simulink model "Servo_model_validate"  (R2020a)
settings: Solver=ode5  StartTime=0.0  StopTime=20  FixedStep=0.002  RelTol=1e-3  AbsTol=1e-6
PreLoadFcn:
  | load servo_chstat
values from neighbouring files (symbols this model uses):
  input_change = 0.07    [lab5.m]
  pwm = [-1 -0.961416361416 -0.923076923077 -0.884493284493 -0.846153846154 -0.80757020757 -0.768986568987 -0.730647130647 -0.692307692308 -0.653724053724 -0.615384615385 -0.576800976801 ... (53 elements, 1x53)]    [servo_chstat.mat]
  vpwm = [-172.202819824 -162.381335449 -154.255700684 -146.997290039 -139.415771484 -132.329187012 -124.019897461 -116.524291992 -108.629003906 -99.2582519531 -92.2202270508 -84.5235351562 ... (53 elements, 1x53)]    [servo_chstat.mat]
libraries: simulink x1
settings Model: ExtModeTrigDuration=12000  ExtModeTrigLevel=0.400000  Creator=jims  LastModifiedBy=ariana
settings SolverCC: AutoScaleAbsTol=off
settings DataIOCC: ExternalInput=[]  InitialState=[]  MaxDataPoints=5000  SaveFormat=Array  SignalLoggingSaveFormat=ModelDataLogs  SaveOutput=off  SaveTime=off  ReturnWorkspaceOutputs=off  SignalLoggingName=sigsOut
settings OptimizationCC: BooleanDataType=off  ExpressionDepthLimit=2147483647  InitFltsAndDblsToZero=on  LifeSpan=inf
settings DebuggingCC: SaveWithParameterizedLinksMsg=none  UnderspecifiedInitializationDetection=Classic  MergeDetectMultiDrivingBlocksExec=none  SignalResolutionControl=TryResolveAllWithWarning  MultiTaskDSMMsg=warning  MultiTaskCondExecSysMsg=none  IntegerOverflowMsg=none  FcnCallInpInsideContextMsg=warning  StateNameClashWarn=warning  SFUnexpectedBacktrackingDiag=warning  SFNoUnconditionalDefaultTransitionDiag=warning  SFExecutionAtInitializationDiag=none  IntegerSaturationMsg=none  ArithmeticOperatorsInVariantConditions=warning
settings HardwareCC: ProdBitPerPointer=32  ProdBitPerSizeT=32  ProdBitPerPtrDiffT=32  ProdLargestAtomicFloat=None  ProdIntDivRoundTo=Undefined  ProdEndianess=Unspecified  ProdWordSize=32  ProdHWDeviceType=32-bit Generic  TargetUnknown=on
settings ModelReferenceCC: PropagateSignalLabelsOutOfModel=off
settings SFSimCC: SimUseLocalCustomCode=off  CustomCodeUndefinedFunction=UseInterfaceOnly
settings RTWCC: SystemTargetFile=rtwin.tlc  TemplateMakefile=rtwintmf  RTWUseLocalCustomCode=off
settings CodeAppCC: StateflowObjectComments=on
settings TargetCC: TargetFcnLib=ansi_tfl_tmw.mat  ModelReferenceCompliant=off  CompOptLevelCompliant=off
settings ConfigComp: CovMetricSettings=dw  CovHtmlReporting=on  CovSaveCumulativeToWorkspaceVar=on  CovSaveSingleToWorkspaceVar=on  CovExternalEMLEnable=off

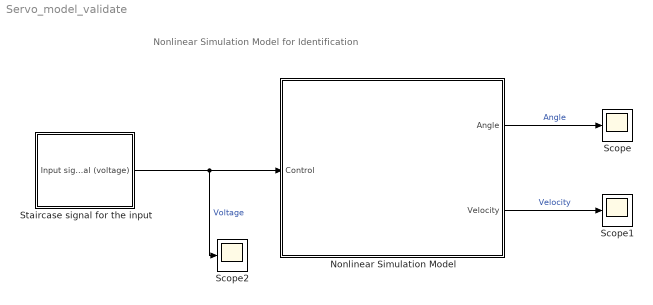
== system Servo_model_validate ==
  note: Nonlinear Simulation Model for Identification
  Nonlinear Simulation Model : Subsystem
  Scope : Scope
  Scope1 : Scope
  Scope2 : Scope
  Staircase signal for the input : Subsystem
  wires:
  Nonlinear Simulation Model/1(Angle) -> Scope/1  "Angle"
  Nonlinear Simulation Model/2(Velocity) -> Scope1/1  "Velocity"
  Staircase signal for the input/1(Input signal (voltage)) -> Scope2/1, Nonlinear Simulation Model/1(Control)  "Voltage"

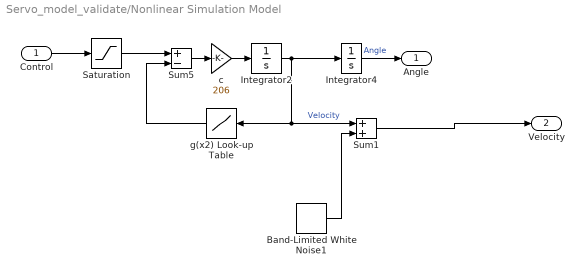
== system Servo_model_validate/Nonlinear Simulation Model ==
  Control : Inport
  Band-Limited White Noise1 : simulink/Sources/Band-Limited White Noise  Cov=[0.001]  Ts=0.02  seed=[23341]
  Integrator2 : Integrator
  Integrator4 : Integrator
  Saturation : Saturate  UpperLimit=1  LowerLimit=-1
  Sum1 : Sum  InputSameDT=on  SaturateOnIntegerOverflow=on  OutDataTypeStr=Inherit: Same as first input
  Sum5 : Sum  Inputs=+-  InputSameDT=on  SaturateOnIntegerOverflow=on  OutDataTypeStr=Inherit: Same as first input
  c : Gain  Gain=206  SaturateOnIntegerOverflow=on  OutDataTypeStr=Inherit: Same as input  ParamDataTypeStr=Inherit: Same as input
  g(x2) Look-up Table : Lookup  InputValues=vpwm  Table=pwm  SaturateOnIntegerOverflow=on
  Angle : Outport  InitialOutput=0  VectorParamsAs1DForOutWhenUnconnected=off
  Velocity : Outport  Port=2  InitialOutput=0  VectorParamsAs1DForOutWhenUnconnected=off
  wires:
  Sum5/1 -> c/1
  g(x2) Look-up Table/1 -> Sum5/2
  Integrator2/1 -> Integrator4/1, g(x2) Look-up Table/1, Sum1/1  "Velocity"
  Integrator4/1 -> Angle/1  "Angle"
  c/1 -> Integrator2/1
  Control/1 -> Saturation/1
  Saturation/1 -> Sum5/1
  Sum1/1 -> Velocity/1
  Band-Limited White Noise1/1 -> Sum1/2

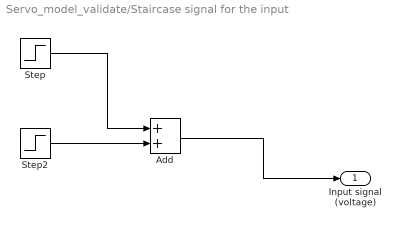
== system Servo_model_validate/Staircase signal for the input ==
  Add : Sum
  Step : Step  Time=0  After=0.4  SampleTime=0
  Step2 : Step  Time=10  After=input_change  SampleTime=0
  Input signal (voltage) : Outport  InitialOutput=0  VectorParamsAs1DForOutWhenUnconnected=off
  wires:
  Step/1 -> Add/1
  Step2/1 -> Add/2
  Add/1 -> Input signal (voltage)/1
